simulink model "state_space"  (R2022b)
settings: Solver=VariableStepAuto  StartTime=0.0  StopTime=10.0  RelTol=1e-3
settings Model: Creator=freshalias  LastModifiedBy=freshalias

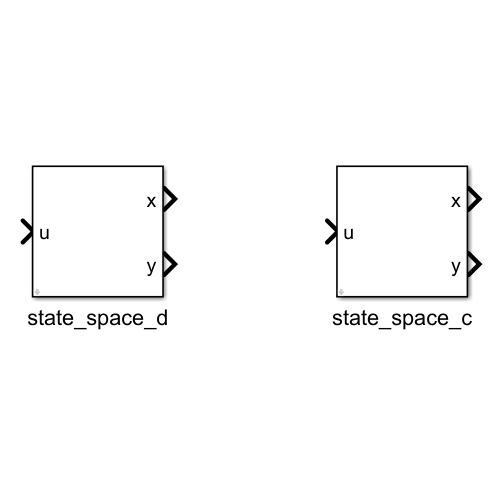
[thumbnail: Simulink's stored preview of the top-level diagram]
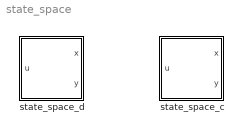
== system state_space ==
  state_space_c : Subsystem  mask{Ac=0, Bc=0, Cc=0, Dc=0, x_0=0}
      mask DialogControl ParameterGroupVar Prompt: 参数
  state_space_d : Subsystem  mask{Ad=0, Bd=0, Cd=0, Dd=0, x_0=0, u_0=0}
      mask DialogControl ParameterGroupVar Prompt: 参数

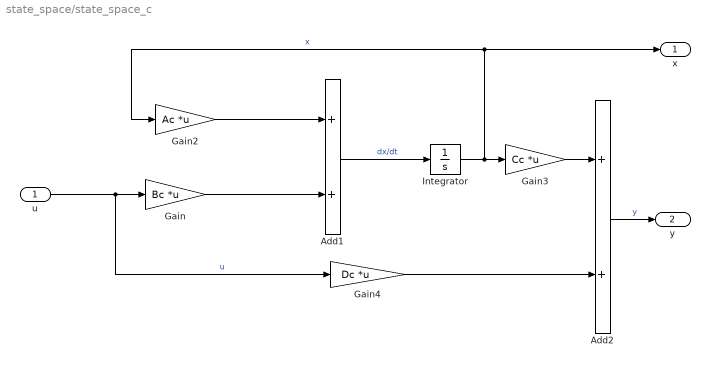
== system state_space/state_space_c ==
  u : Inport
  Add1 : Sum
  Add2 : Sum
  Gain : Gain  Gain=Bc  Multiplication=Matrix(K*u)
  Gain2 : Gain  Gain=Ac  Multiplication=Matrix(K*u)
  Gain3 : Gain  Gain=Cc  Multiplication=Matrix(K*u)
  Gain4 : Gain  Gain=Dc  Multiplication=Matrix(K*u)
  Integrator : Integrator  InitialCondition=x_0
  x : Outport
  y : Outport  Port=2
  wires:
  Gain2/1 -> Add1/1
  Gain/1 -> Add1/2
  Add1/1 -> Integrator/1  "dx/dt"
  Integrator/1 -> Gain3/1, Gain2/1, x/1  "x"
  u/1 -> Gain/1, Gain4/1  "u"
  Gain3/1 -> Add2/1
  Gain4/1 -> Add2/2
  Add2/1 -> y/1  "y"

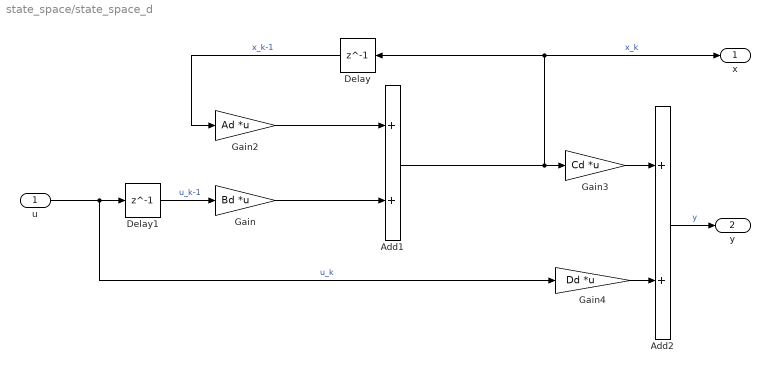
== system state_space/state_space_d ==
  u : Inport
  Add1 : Sum
  Add2 : Sum
  Delay : Delay  DelayLength=1  InitialCondition=x_0
  Delay1 : Delay  DelayLength=1  InitialCondition=u_0
  Gain : Gain  Gain=Bd  Multiplication=Matrix(K*u)
  Gain2 : Gain  Gain=Ad  Multiplication=Matrix(K*u)
  Gain3 : Gain  Gain=Cd  Multiplication=Matrix(K*u)
  Gain4 : Gain  Gain=Dd  Multiplication=Matrix(K*u)
  x : Outport
  y : Outport  Port=2
  wires:
  Gain2/1 -> Add1/1
  Gain/1 -> Add1/2
  Add1/1 -> Gain3/1, Delay/1, x/1  "x_k"
  Gain3/1 -> Add2/1
  Gain4/1 -> Add2/2
  Add2/1 -> y/1  "y"
  u/1 -> Gain4/1, Delay1/1  "u_k"
  Delay1/1 -> Gain/1  "u_k-1"
  Delay/1 -> Gain2/1  "x_k-1"
